simulink model "CMD_LPF_CUTOFF_Test"  (R2024a)
settings: Solver=VariableStepAuto  StartTime=0.0  StopTime=10.0  RelTol=1e-3
libraries: simulink x5, cstblocks x2
settings Model: Creator=UASG  LastModifiedBy=UASG

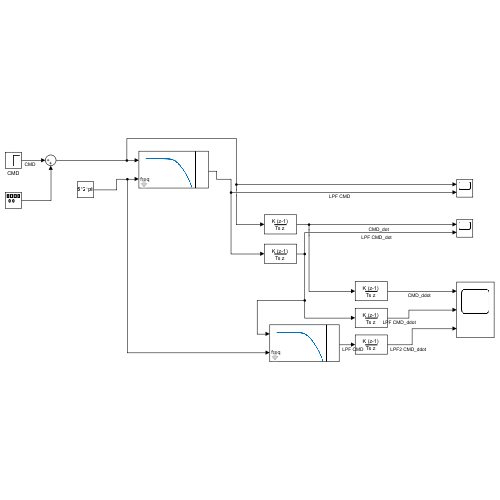
[thumbnail: Simulink's stored preview of the top-level diagram]
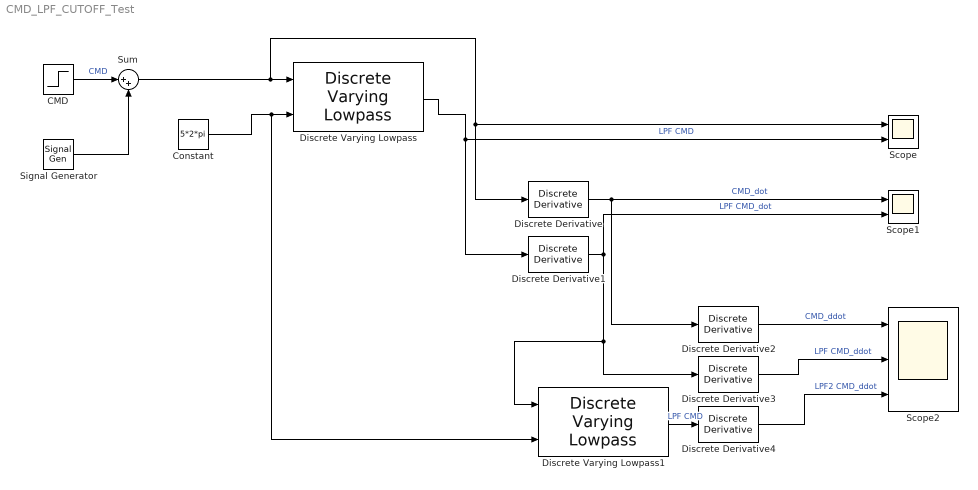
== system CMD_LPF_CUTOFF_Test ==
  CMD : Step  SampleTime=1/250
  Constant : Constant  Value=5*2*pi  SampleTime=1/250
  Discrete Derivative{,1..4} (5 alike) : simulink/Discrete/Discrete Derivative  gainval=1.0  ICPrevScaledInput=0.0  OutMin=[]  OutMax=[]  OutDataType=fixdt(1, 16)  OutScaling=2^-10  DoSatur=off
  Discrete Varying Lowpass : cstblocks/Linear Parameter Varying/Discrete Varying Lowpass  N=1  w0=0  Ts=1/250
  Discrete Varying Lowpass1 : cstblocks/Linear Parameter Varying/Discrete Varying Lowpass  N=1  w0=0  Ts=1/250
  Scope : Scope  NumInputPorts=2
  Scope1 : Scope  NumInputPorts=2
  Scope2 : Scope  NumInputPorts=3
  Signal Generator : SignalGenerator  Amplitude=0.5  Frequency=1*2*pi  Units=rad/sec
  Sum : Sum  Inputs=|++
  wires:
  Discrete Varying Lowpass/1 -> Discrete Derivative1/1, Scope/2  "LPF CMD"
  Constant/1 -> Discrete Varying Lowpass1/2, Discrete Varying Lowpass/2
  Discrete Derivative/1 -> Discrete Derivative2/1, Scope1/1  "CMD_dot"
  Discrete Derivative1/1 -> Discrete Varying Lowpass1/1, Discrete Derivative3/1, Scope1/2  "LPF CMD_dot"
  Discrete Derivative2/1 -> Scope2/1  "CMD_ddot"
  Discrete Derivative3/1 -> Scope2/2  "LPF CMD_ddot"
  Discrete Varying Lowpass1/1 -> Discrete Derivative4/1  "LPF CMD"
  Discrete Derivative4/1 -> Scope2/3  "LPF2 CMD_ddot"
  CMD/1 -> Sum/1  "CMD"
  Sum/1 -> Discrete Derivative/1, Scope/1, Discrete Varying Lowpass/1
  Signal Generator/1 -> Sum/2
